simulink model "DcMotorReverseSpeed"  (R2018a)
settings: Solver=VariableStepAuto  StartTime=0.0  StopTime=10.0  RelTol=1e-3
libraries: powerlib x8
settings Model: Creator=Bhaskar  LastModifiedBy=Bhaskar

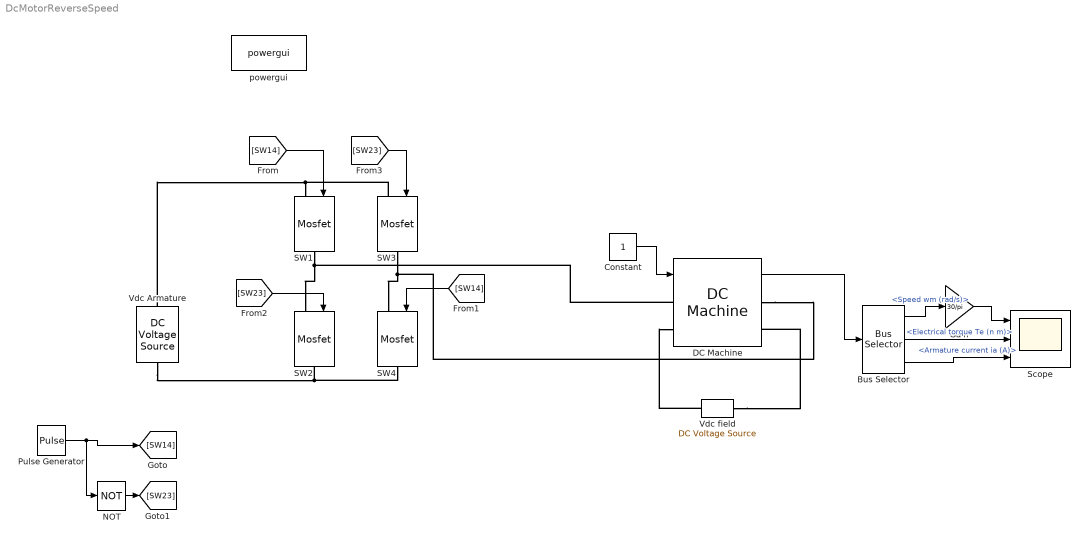
== system DcMotorReverseSpeed ==
  Bus Selector : BusSelector  OutputSignals=Speed wm (rad/s),Electrical torque Te (n m),Armature current ia (A)
  Constant : Constant
  DC Machine : powerlib/Machines/DC Machine  PresetModel=01: 5HP 240V 1750RPM Field:300V  MechanicalLoad=Torque TL  FieldType=Wound  ShowDetailedParameters=on  MeasurementBus=off  RLa=[2.581 0.028]  RLf=[281.3 156]  Laf=0.9483  MachineConstant=Torque constant (N.m/A)  Ke=1.8  Kt=1.8  J=0.02215  Bm=0.002953  Tf=0.5161  w0=1  Ifinit=1  TsPowergui=0  TsBlock=-1
  Gain : Gain  Gain=30/pi
  NOT : Logic  Operator=NOT  IconShape=distinctive  AllPortsSameDT=off  OutDataTypeStr=boolean
  Pulse Generator : DiscretePulseGenerator  PulseType=Time based  Period=1/1000  PulseWidth=25
  SW{1..4} (4 alike) : powerlib/Power Electronics/Mosfet  Ron=0.1  Lon=0  Rd=0.01  Vfd=0  IC=0  Rs=1e5  Cs=inf  Measurements=off
  Scope : Scope  NumInputPorts=3
  Vdc Armature : powerlib/Electrical Sources/DC Voltage Source  Amplitude=240  Measurements=None
  "Vdc field " : powerlib/Electrical Sources/DC Voltage Source  Amplitude=300  Measurements=None
  powergui : powerlib/powergui  Priority=1  SimulationMode=Discrete  SampleTime=50e-6  frequency=60  Iterations=50  frequencyindice=0  Pbase=100e6  ErrMax=1e-4  UnitsV=kV  UnitsW=MW  buscounter=0  FunctionMessages=off  echomessages=off  EnableUseOfTLC=off  CurrentSourceSwitches=off  DisableSnubberDevices=off  DisableRonSwitches=off  DisableVfSwitches=off  DisplayEquations=off  SolverType=Tustin/Backward Euler (TBE)  Interpol=off  ExternalGateDelay=off  methode=off  Ts=100  x0status=blocks  SPID=on  SwTol=0  HookPort=off  RestoreLinks=warning  ResistiveCurrentMeasurement=off  Frange=[0:2:500]  Ylog=off  Xlog=on  ShowGrid=off  save=off  variable=ZData  structure=0  ZoomFFT=off  StartTime=0.0  cycles=1  DisplayStyle=1  fundamental=60  FreqAxis=off  MaxFrequency=1000  frequencyindicesteady=1  RmsSteady=1  display=off
  wires:
  DC Machine/1 -> Bus Selector/1
  [SW23] -> SW2/1
  Bus Selector/3 -> Scope/3  "<Armature current ia (A)>"
  Bus Selector/2 -> Scope/2  "<Electrical torque Te (n m)>"
  Gain/1 -> Scope/1
  Constant/1 -> DC Machine/1
  [SW14] -> SW1/1
  NOT/1 -> [SW23]
  Bus Selector/1 -> Gain/1  "<Speed wm (rad/s)>"
  [SW14] -> SW4/1
  [SW23] -> SW3/1
  Pulse Generator/1 -> NOT/1, [SW14]
  connections:
  SW3/RConn1 -- DC Machine/RConn1 -- SW4/LConn1
  SW2/RConn1 -- Vdc Armature/LConn1 -- SW4/RConn1
  SW1/LConn1 -- Vdc Armature/RConn1 -- SW3/LConn1
  SW1/RConn1 -- DC Machine/LConn1 -- SW2/LConn1
  "Vdc field "/LConn1 -- DC Machine/RConn2
  "Vdc field "/RConn1 -- DC Machine/LConn2
